simulink library "PowerFlowLib"  (R2015b)
settings: Solver=ode45  StartTime=0.0  StopTime=10.0  RelTol=1e-3
undefined symbols (not defined in the file or in its folder): Air, AirProp, C, F1, F2, Fanmap, Fld1, Fld2, Fluid, fueltankdata, HydProp, HydraulicLoad, IBFD_exc, L, LoadFluidProps, magnitude, MSSN, n_alghts, PumpProp, pwr_alghts, R_fd_exc, Rcore, Ts, VBFD_exc
libraries: PowerFlowLib x35, simulink x19, powerlib_extras x2, dspstat3 x2
(part 12 of 12)

== system PowerFlowLib/Energy & Power Systems/Electrical/Battery/BATTERY/SINGLE CELL VOLT OUT/CHARGE/RCh ==
  SOC : Inport
  current : Inport  Port=2
  Add1 : Sum  Inputs=+-
  Ch : Fcn  Expr=493923+3e7*u-1e8*u^2+2e8*u^3-9e7*u^4
  Integrator2 : Integrator
  Math Function : Math  Operator=reciprocal  SaturateOnIntegerOverflow=on
  Math Function1 : Math  Operator=reciprocal  SaturateOnIntegerOverflow=on
  Product1 : Product  RndMeth=Zero
  Product2 : Product  RndMeth=Zero
  Rh : Fcn  Expr=0.1484-1.1978*u+3.5946*u^2-4.3618*u^3+1.8335*u^4
  Drop : Outport
  Rh_Charge : Outport  Port=2
  wires:
  Rh/1 -> Math Function/1, Rh_Charge/1
  current/1 -> Add1/1
  Product1/1 -> Add1/2
  Math Function/1 -> Product1/2
  Integrator2/1 -> Product1/1, Drop/1
  Ch/1 -> Math Function1/1
  Add1/1 -> Product2/1
  Math Function1/1 -> Product2/2
  Product2/1 -> Integrator2/1
  SOC/1 -> Ch/1, Rh/1

== system PowerFlowLib/Energy & Power Systems/Electrical/Battery/BATTERY/SINGLE CELL VOLT OUT/CHARGE/RCm ==
  SOC : Inport
  current : Inport  Port=2
  Add1 : Sum  Inputs=+-
  Cm_C : Fcn  Expr=216.52+28308*u-166348*u^2+431168*u^3-491497*u^4+199631*u^5
  Integrator2 : Integrator
  Math Function : Math  Operator=reciprocal  SaturateOnIntegerOverflow=on
  Math Function1 : Math  Operator=reciprocal  SaturateOnIntegerOverflow=on
  Product1 : Product  RndMeth=Zero
  Product2 : Product  RndMeth=Zero
  Rm_C : Fcn  Expr=1.83-35.02*u+246.62*u^2-785.59*u^3+1250.7*u^4-970.92*u^5+292.72*u^6
  Drop : Outport
  Rm_Charge : Outport  Port=2
  wires:
  Rm_C/1 -> Math Function/1, Rm_Charge/1
  current/1 -> Add1/1
  Product1/1 -> Add1/2
  Math Function/1 -> Product1/2
  Integrator2/1 -> Product1/1, Drop/1
  Cm_C/1 -> Math Function1/1
  Add1/1 -> Product2/1
  Math Function1/1 -> Product2/2
  Product2/1 -> Integrator2/1
  SOC/1 -> Rm_C/1, Cm_C/1

== system PowerFlowLib/Energy & Power Systems/Electrical/Battery/BATTERY/SINGLE CELL VOLT OUT/CHARGE/RCs ==
  SOC : Inport
  current : Inport  Port=2
  Add1 : Sum  Inputs=+-
  Cs_C : Fcn  Expr=0.9936+14.521*u-91.975*u^2+199*u^3-179.67*u^4+57.922*u^5
  Integrator2 : Integrator
  Math Function : Math  Operator=reciprocal  SaturateOnIntegerOverflow=on
  Math Function1 : Math  Operator=reciprocal  SaturateOnIntegerOverflow=on
  Product1 : Product  RndMeth=Zero
  Product2 : Product  RndMeth=Zero
  Rs_C : Fcn  Expr=0.1135-0.9797*u+5.1623*u^2-11.47*u^3+11.125*u^4-3.9253*u^5
  Drop : Outport
  Rs_Charge : Outport  Port=2
  wires:
  Rs_C/1 -> Math Function/1, Rs_Charge/1
  current/1 -> Add1/1
  Product1/1 -> Add1/2
  Math Function/1 -> Product1/2
  Integrator2/1 -> Product1/1, Drop/1
  Cs_C/1 -> Math Function1/1
  Add1/1 -> Product2/1
  Math Function1/1 -> Product2/2
  Product2/1 -> Integrator2/1
  SOC/1 -> Rs_C/1, Cs_C/1

== system PowerFlowLib/Energy & Power Systems/Electrical/Battery/BATTERY/SINGLE CELL VOLT OUT/DISCHARGE/RCh ==
  SOC : Inport
  current : Inport  Port=2
  Add1 : Sum  Inputs=+-
  Ch : Fcn  Expr=493923+3e7*u-1e8*u^2+2e8*u^3-9e7*u^4
  Integrator2 : Integrator
  Math Function : Math  Operator=reciprocal  SaturateOnIntegerOverflow=on
  Math Function1 : Math  Operator=reciprocal  SaturateOnIntegerOverflow=on
  Product1 : Product  RndMeth=Zero
  Product2 : Product  RndMeth=Zero
  Rh : Fcn  Expr=0.1484-1.1978*u+3.5946*u^2-4.3618*u^3+1.8335*u^4
  Drop : Outport
  Rh_Dchg : Outport  Port=2
  wires:
  SOC/1 -> Rh/1, Ch/1
  Product2/1 -> Integrator2/1
  Math Function1/1 -> Product2/2
  Add1/1 -> Product2/1
  Ch/1 -> Math Function1/1
  Integrator2/1 -> Product1/1, Drop/1
  Math Function/1 -> Product1/2
  Product1/1 -> Add1/2
  current/1 -> Add1/1
  Rh/1 -> Math Function/1, Rh_Dchg/1

== system PowerFlowLib/Energy & Power Systems/Electrical/Battery/BATTERY/SINGLE CELL VOLT OUT/DISCHARGE/RCm ==
  SOC : Inport
  current1 : Inport  Port=2
  Add1 : Sum  Inputs=+-
  Cm : Fcn  Expr=239.49-14755*u+264236*u^2-825025*u^3+947250*u^4-371150*u^5
  Integrator3 : Integrator
  Math Function : Math  Operator=reciprocal  SaturateOnIntegerOverflow=on
  Math Function1 : Math  Operator=reciprocal  SaturateOnIntegerOverflow=on
  Product2 : Product  RndMeth=Zero
  Product3 : Product  RndMeth=Zero
  Rm : Fcn  Expr=1.95-33.837*u+228.96*u^2-712.75*u^3+1118.1*u^4-859.2*u^5+257.11*u^6
  Drop : Outport
  Rm_Dchg : Outport  Port=2
  wires:
  Rm/1 -> Math Function/1, Rm_Dchg/1
  current1/1 -> Add1/1
  Product2/1 -> Add1/2
  Math Function/1 -> Product2/2
  Integrator3/1 -> Product2/1, Drop/1
  Cm/1 -> Math Function1/1
  Add1/1 -> Product3/1
  Math Function1/1 -> Product3/2
  Product3/1 -> Integrator3/1
  SOC/1 -> Rm/1, Cm/1

== system PowerFlowLib/Energy & Power Systems/Electrical/Battery/BATTERY/SINGLE CELL VOLT OUT/DISCHARGE/RCs ==
  SOC : Inport
  current : Inport  Port=2
  Add1 : Sum  Inputs=+-
  Cs : Fcn  Expr=0.7472+9.0675*u-30.712*u^2+32.551*u^3-7.358*u^4-3.4621*u^5
  Integrator2 : Integrator
  Math Function : Math  Operator=reciprocal  SaturateOnIntegerOverflow=on
  Math Function1 : Math  Operator=reciprocal  SaturateOnIntegerOverflow=on
  Product1 : Product  RndMeth=Zero
  Product2 : Product  RndMeth=Zero
  Rs : Fcn  Expr=0.1457-1.0586*u+4.867*u^2-10.131*u^3+9.5077*u^4-3.3024*u^5
  Drop : Outport
  Rs_Dchg : Outport  Port=2
  wires:
  Rs/1 -> Math Function/1, Rs_Dchg/1
  current/1 -> Add1/1
  Product1/1 -> Add1/2
  Math Function/1 -> Product1/2
  Integrator2/1 -> Product1/1, Drop/1
  Cs/1 -> Math Function1/1
  Add1/1 -> Product2/1
  Math Function1/1 -> Product2/2
  Product2/1 -> Integrator2/1
  SOC/1 -> Rs/1, Cs/1

== system PowerFlowLib/Energy & Power Systems/Thermal/ECS/Air-Air HX/HX_and_Fin_paramters/HX_parameters/Calculating the no of passages per fluid flow ==
  Raw_HX_parameters : Inport
  Fin_parameters : Inport  Port=2
  Add : Sum  Inputs=+---
  Add1 : Sum  Inputs=+++
  Bus Selector : BusSelector  OutputSignals=H_hx,t_p
  Bus Selector1 : BusSelector  OutputSignals=h_fin,t_fin
  Display : Display
  Divide : Product  Inputs=*/
  Gain{,1..3} (4 alike) : Gain  Gain=2
  Rounding Function : Rounding  Operator=round
  N_passages_per_flow : Outport
  wires:
  Rounding Function/1 -> Display/1, N_passages_per_flow/1
  Divide/1 -> Rounding Function/1
  Add1/1 -> Divide/2
  Add/1 -> Divide/1
  Gain3/1 -> Add1/3
  Gain2/1 -> Add1/2
  Gain1/1 -> Add1/1
  Gain/1 -> Add/4
  Bus Selector/2 -> Gain3/1, Gain/1  "<t_p>"
  Bus Selector1/2 -> Gain2/1, Add/3  "<t_fin>"
  Bus Selector1/1 -> Gain1/1, Add/2  "<h_fin>"
  Bus Selector/1 -> Add/1  "<H_hx>"
  Fin_parameters/1 -> Bus Selector1/1
  Raw_HX_parameters/1 -> Bus Selector/1

== system PowerFlowLib/Energy & Power Systems/Thermal/ECS/Air-Air HX/HX_and_Fin_paramters/HX_parameters/Calculating the total number of fins per HX per fluid flow ==
  Raw_HX_parameters : Inport
  Fin_parameters : Inport  Port=2
  N_passages_per_flow : Inport  Port=3
  Bus Selector : BusSelector  OutputSignals=W_hx,L_hx
  Bus Selector1 : BusSelector  OutputSignals=s_fin,t_fin,l_fin
  Divide : Product  Inputs=***//
  Rounding Function : Rounding  Operator=round
  s+t : Sum
  Tot_no_of_fins_per_HX_per_flow : Outport
  wires:
  Rounding Function/1 -> Tot_no_of_fins_per_HX_per_flow/1
  Divide/1 -> Rounding Function/1
  Bus Selector1/3 -> Divide/5  "<l_fin>"
  s+t/1 -> Divide/4  "s+t"
  N_passages_per_flow/1 -> Divide/3
  Bus Selector/2 -> Divide/2  "<L_hx>"
  Bus Selector/1 -> Divide/1  "<W_hx>"
  Bus Selector1/2 -> s+t/2  "<t_fin>"
  Bus Selector1/1 -> s+t/1  "<s_fin>"
  Fin_parameters/1 -> Bus Selector1/1
  Raw_HX_parameters/1 -> Bus Selector/1

== system PowerFlowLib/Energy & Power Systems/Thermal/ECS/Air-Air HX/HX_and_Fin_paramters/HX_parameters/Calculating total free flow area per flow ==
  Raw_HX_parameters : Inport
  Fin_parameters : Inport  Port=2
  N_passages_per_flow : Inport  Port=3
  "Calculating the per fin ratio of the free flow area to the frontal area " : Subsystem
  Calculating total passages area per flow : Subsystem
  Product : Product  RndMeth=Zero
  Total_free_flow_area : Outport
  wires:
  Product/1 -> Total_free_flow_area/1
  Calculating total passages area per flow/1(total_pasages_area_per_flow) -> Product/2
  "Calculating the per fin ratio of the free flow area to the frontal area "/1(Per fin ratio of the free flow to the frontal areas) -> Product/1
  N_passages_per_flow/1 -> Calculating total passages area per flow/3(N_passages_per_flow)
  Raw_HX_parameters/1 -> Calculating total passages area per flow/2("HX_parameters ")
  Fin_parameters/1 -> Calculating total passages area per flow/1(Fin_parameters), "Calculating the per fin ratio of the free flow area to the frontal area "/1(Fin_parameters)

== system PowerFlowLib/Energy & Power Systems/Thermal/ECS/Air-Air HX/HX_and_Fin_paramters/HX_parameters/Calculating total free flow area per flow/Calculating the per fin ratio of the free flow area to the frontal area  ==
  Fin_parameters : Inport
  Bus Selector1 : BusSelector  OutputSignals=s_fin,t_fin,h_fin
  Divide : Product  Inputs=**//
  h+t : Sum
  s+t : Sum
  s-t : Sum  Inputs=+-
  Per fin ratio of the free flow to the frontal areas : Outport
  wires:
  Divide/1 -> Per fin ratio of the free flow to the frontal areas/1
  h+t/1 -> Divide/4  "h+t"
  s+t/1 -> Divide/3  "s+t"
  s-t/1 -> Divide/1  "s-t"
  Bus Selector1/3 -> Divide/2, h+t/2  "<h_fin>"
  Bus Selector1/2 -> h+t/1, s+t/2, s-t/2  "<t_fin>"
  Bus Selector1/1 -> s+t/1, s-t/1  "<s_fin>"
  Fin_parameters/1 -> Bus Selector1/1

== system PowerFlowLib/Energy & Power Systems/Thermal/ECS/Air-Air HX/HX_and_Fin_paramters/HX_parameters/Calculating total free flow area per flow/Calculating total passages area per flow ==
  Fin_parameters : Inport
  "HX_parameters " : Inport  Port=2
  N_passages_per_flow : Inport  Port=3
  Bus Selector : BusSelector  OutputSignals=h_fin,t_fin
  Bus Selector1 : BusSelector  OutputSignals=W_hx
  Divide : Product  Inputs=***
  h+t : Sum
  total_pasages_area_per_flow : Outport
  wires:
  Divide/1 -> total_pasages_area_per_flow/1
  Bus Selector1/1 -> Divide/2  "<W_hx>"
  h+t/1 -> Divide/1
  Bus Selector/2 -> h+t/2  "<t_fin>"
  Bus Selector/1 -> h+t/1  "<h_fin>"
  N_passages_per_flow/1 -> Divide/3
  "HX_parameters "/1 -> Bus Selector1/1
  Fin_parameters/1 -> Bus Selector/1

== matlab function PowerFlowLib/Energy & Power Systems/Hydraulic/Hydraulic Load/MATLAB Function ==
  data: phase_id output; prev_phase input; y output; curr_phase input
function [phase_id,y] = fcn(prev_phase,curr_phase)
%#codegen

% phase identification numbers are set via the mission profile block
% they are as follows:
% 1: startup 2: taxi 3: takeoff 4: climb 5: cruise 6: descent
% 7: loiter 8: approach 9: landing 10: landing taxi 11: shutdown 12: idle 
phase_id = curr_phase;

% checking for phase switch
% on a flight phase switch, y is pulsed low then high
% this resets the timer counter that is input to the 2D lookup table
% for the hydraulic loads
for i = 1:size(prev_phase,2)
    if prev_phase(i) ~= curr_phase(i)
        y = 0;
    else
        y = 1;
    end
end

== matlab function PowerFlowLib/Energy & Power Systems/Thermal/Fuel & Oil/Fluid Tank/Warning msg/MATLAB Function ==
  data: y output; time input
function y = fcn(time)
coder.extrinsic('warning')
coder.extrinsic('gcb')
coder.extrinsic('num2str')
blk = gcb;
blk = strrep(blk,'/Warning msg/MATLAB Function/ SFunction','');
warning([blk,'is empty at ',num2str(time),' seconds. Mass flow rate out has been set to 0 for all time after.']);

y = 0;
